simulink model "iron_filter0"  (Simulink 8.5)
settings: Solver=ode15s  StartTime=0.0  StopTime=2*24*3600
undefined symbols (not defined in the file or in its folder): B, U, x0
settings Model: Creator=M.Sparnaaij  LastModifiedBy=Martijn  ExtModeTrigMode=oneshot  ExtModeArmWhenConnect=off
settings DataIOCC: LimitDataPoints=off  SignalLoggingName=sigsOut
settings OptimizationCC: BooleanDataType=off
settings DebuggingCC: SaveWithParameterizedLinksMsg=none  SignalResolutionControl=TryResolveAllWithWarning  MultiTaskDSMMsg=warning  MultiTaskCondExecSysMsg=none  FcnCallInpInsideContextMsg=EnableAllAsWarning  StrictBusMsg=None
settings HardwareCC: TargetUnknown=on

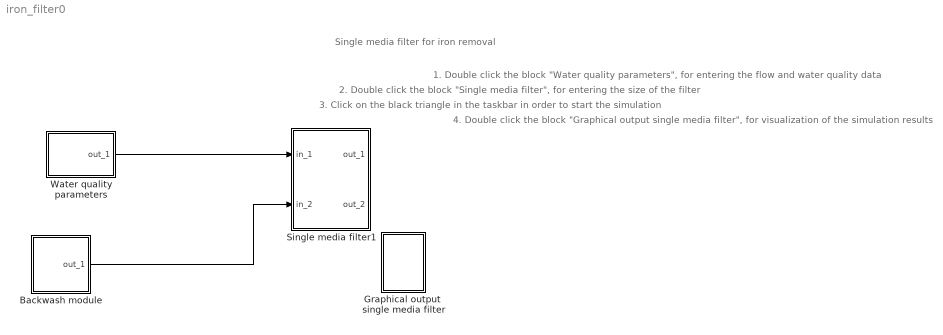
== system iron_filter0 ==
  note: Single media filter for iron removal
  note: 2. Double click the block "Single media filter", for entering the size of the filter
  note: 3. Click on the black triangle in the taskbar in order to start the simulation
  note: 4. Double click the block "Graphical output single media filter", for visualization of the simulation results
  note: 1. Double click the block "Water quality parameters", for entering the flow and water quality data
  Backwash module : Subsystem  Description=During a simulation the filter can be backwashed with the backwash module, so a number of successive filterruns can be simulated.
      mask init:
      | filenaam='./Backwash_module.mat';
      | 
      | errstr = st_UniqName(filenaam,'filenaam=''','SubSystem','OpenFcn');
      | if errstr, error([errstr 'The filename "' filenaam '" is already in use. Choose a different filename.']), end
      | 
      | P = bacwa1_p(filenaam);
      | [B,x0,U]=bacwa1_i(filenaam);
      settings: OpenFcn=|
      | filenaam='./Backwash_module.mat';
      | st_ParameterInput('init',gcb,filenaam,'bacwa1');
      mask Display:
      | plot(0,0,100,100,[80,80,20,20],[80,20,20,80],[40,42,38,40,40],[70,67,67,70,30],[60,62,58,60,60],[70,67,67,70,30])
      | disp('')
      | text(50,50,'bacwa1', 'horizontalAlignment', 'center', 'verticalAlignment', 'middle');
      | text(0,0,filenaam, 'horizontalAlignment', 'left', 'verticalAlignment', 'bottom');
  Graphical output  single media filter : Subsystem
      settings: OpenFcn=irofil_g
      mask Display:
      | plot(0,0,100,100,[80,20,20],[20,20,80],[80,69,60,52,45,39,33,28,24,20],[65,65,64,61,57,52,45,37,30,20])
      | disp('');
      | text(100,100,'irofil', 'horizontalAlignment', 'right', 'verticalAlignment', 'top');
  Single media filter1 : Subsystem  Description=This model calculates the removal of suspended solids with a single media filter.
      mask init:
      | filenaam='./Single_media_filter1.mat';
      | 
      | errstr = st_UniqName(filenaam,'filenaam=''','SubSystem','OpenFcn');
      | if errstr, error([errstr 'The filename "' filenaam '" is already in use. Choose a different filename.']), end
      | 
      | P = irofil_p(filenaam);
      | [B,x0,U]=irofil_i(filenaam);
      settings: OpenFcn=|
      | filenaam='./Single_media_filter1.mat';
      | st_ParameterInput('init',gcb,filenaam,'irofil');
      mask Display:
      | plot(0,0,100,100,[25.000000,25.000000,75.000000,75.000000,87.500000],[75.000000,25.000000,25.000000,30.000000,30.000000],[87.500000,75.000000,75.000000],[37.500000,37.500000,75.000000],[25.000000,75.000000],[65.000000,65.000000],[25.000000,75.000000],[42.500000,42.500000],[37.500000,42.500000],[52.500000,52.500000],[50.000000,55.000000],[52.500000,52.500000],[62.500000,67.500000],[52.500000,52.500000])
      | disp('')
      | text(50,50,'irofil', 'horizontalAlignment', 'center', 'verticalAlignment', 'middle');
      | text(0,0,filenaam, 'horizontalAlignment', 'left', 'verticalAlignment', 'bottom');
  Water quality parameters : Subsystem  Description=The water flow and the water quality data must be filled out in the 'Water quality parameters' block. Each project must start with a 'Water quality parameters' block.
      mask init:
      | filenaam='./Water_qual_param.mat';
      | 
      | errstr = st_UniqName(filenaam,'filenaam=''','SubSystem','OpenFcn');
      | if errstr, error([errstr 'The filename "' filenaam '" is already in use. Choose a different filename.']), end
      | 
      | P = invruw_p(filenaam);
      | [B,x0,U]=invruw_i(filenaam);
      settings: OpenFcn=|
      | filenaam='./Water_qual_param.mat';
      | st_ParameterInput('init',gcb,filenaam,'invruw');
      mask Display:
      | plot(0,0,100,100,[80 100],[ 50 50],[20 80 80 20 20],[10 10 90  90 10]);disp('')
      | text(50,50,'invruw', 'horizontalAlignment', 'center', 'verticalAlignment', 'middle');
      | text(0,0,filenaam, 'horizontalAlignment', 'left', 'verticalAlignment', 'bottom');
  wires:
  Water quality parameters/1(out_1) -> Single media filter1/1(in_1)
  Backwash module/1(out_1) -> Single media filter1/2(in_2)

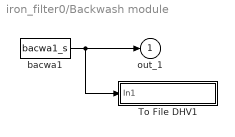
== system iron_filter0/Backwash module ==
  To File DHV1 : Subsystem  mask(To File DHV){naam=[filenaam(1:length(filenaam)-4) '_out.sti']}
      mask prompts: naam "Naam van bestand"
      mask init:
      | set_param([gcb '/To File'],'Filename',naam);
      mask Display: disp(naam)
  bacwa1 : S-Function  FunctionName=bacwa1_s  Parameters=B,x0,U,P
  out_1 : Outport  InitialOutput=0
  wires:
  bacwa1/1 -> To File DHV1/1(In1), out_1/1

== system iron_filter0/Graphical output  single media filter ==
  note: plotten

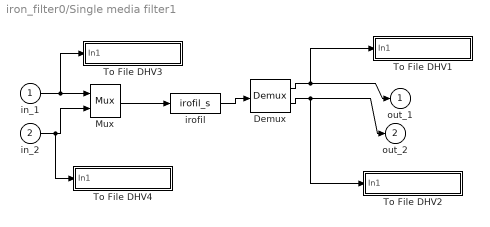
== system iron_filter0/Single media filter1 ==
  in_1 : Inport
  in_2 : Inport  Port=2
  Demux : Demux  Outputs=[U.Number B.Measurements]
  Mux : Mux  Inputs=[U.Number B.Setpoints]
  To File DHV1 : Subsystem  mask(To File DHV){naam=[filenaam(1:length(filenaam)-4) '_out.sti']}
      mask prompts: naam "Naam van bestand"
      mask init:
      | set_param([gcb '/To File'],'Filename',naam);
      mask Display: disp(naam)
  To File DHV2 : Subsystem  mask(To File DHV){naam=[filenaam(1:length(filenaam)-4) '_EM.sti']}
      mask prompts: naam "Naam van bestand"
      mask init:
      | set_param([gcb '/To File'],'Filename',naam);
      mask Display: disp(naam)
  To File DHV3 : Subsystem  mask(To File DHV){naam=[filenaam(1:length(filenaam)-4) '_in.sti']}
      mask prompts: naam "Naam van bestand"
      mask init:
      | set_param([gcb '/To File'],'Filename',naam);
      mask Display: disp(naam)
  To File DHV4 : Subsystem  mask(To File DHV){naam=[filenaam(1:length(filenaam)-4) '_ES.sti']}
      mask prompts: naam "Naam van bestand"
      mask init:
      | set_param([gcb '/To File'],'Filename',naam);
      mask Display: disp(naam)
  irofil : S-Function  FunctionName=irofil_s  Parameters=B,x0,U,P
  out_1 : Outport  InitialOutput=0
  out_2 : Outport  Port=2  InitialOutput=0
  wires:
  in_2/1 -> To File DHV4/1(In1), Mux/2
  Mux/1 -> irofil/1
  in_1/1 -> To File DHV3/1(In1), Mux/1
  irofil/1 -> Demux/1
  Demux/1 -> To File DHV1/1(In1), out_1/1
  Demux/2 -> To File DHV2/1(In1), out_2/1

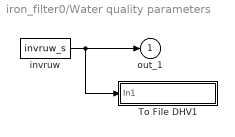
== system iron_filter0/Water quality parameters ==
  To File DHV1 : Subsystem  mask(To File DHV){naam=[filenaam(1:length(filenaam)-4) '_out.sti']}
      mask prompts: naam "Naam van bestand"
      mask init:
      | set_param([gcb '/To File'],'Filename',naam);
      mask Display: disp(naam)
  invruw : S-Function  FunctionName=invruw_s  Parameters=B,x0,U,P
  out_1 : Outport  InitialOutput=0
  wires:
  invruw/1 -> To File DHV1/1(In1), out_1/1

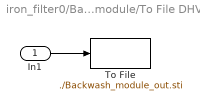
== system iron_filter0/Backwash module/To File DHV1 ==
  In1 : Inport
  To File : ToFile  Filename=./Backwash_module_out.sti  MatrixName=bacwa1out
  wires:
  In1/1 -> To File/1

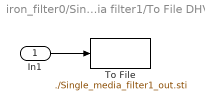
== system iron_filter0/Single media filter1/To File DHV1 ==
  In1 : Inport
  To File : ToFile  Filename=./Single_media_filter1_out.sti  MatrixName=irofilout
  wires:
  In1/1 -> To File/1

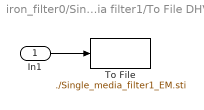
== system iron_filter0/Single media filter1/To File DHV2 ==
  In1 : Inport
  To File : ToFile  Filename=./Single_media_filter1_EM.sti  MatrixName=irofilEM
  wires:
  In1/1 -> To File/1

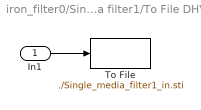
== system iron_filter0/Single media filter1/To File DHV3 ==
  In1 : Inport
  To File : ToFile  Filename=./Single_media_filter1_in.sti  MatrixName=irofilin
  wires:
  In1/1 -> To File/1

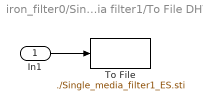
== system iron_filter0/Single media filter1/To File DHV4 ==
  In1 : Inport
  To File : ToFile  Filename=./Single_media_filter1_ES.sti  MatrixName=irofilES
  wires:
  In1/1 -> To File/1

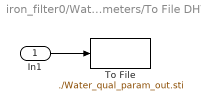
== system iron_filter0/Water quality parameters/To File DHV1 ==
  In1 : Inport
  To File : ToFile  Filename=./Water_qual_param_out.sti  MatrixName=invruwout
  wires:
  In1/1 -> To File/1
